simulink model "Dynamic"  (R2016b)
settings: Solver=ode4  StartTime=0.0  StopTime=13.7777  FixedStep=0.01  RelTol=1e-3
settings Model: Creator=Admin  LastModifiedBy=HP

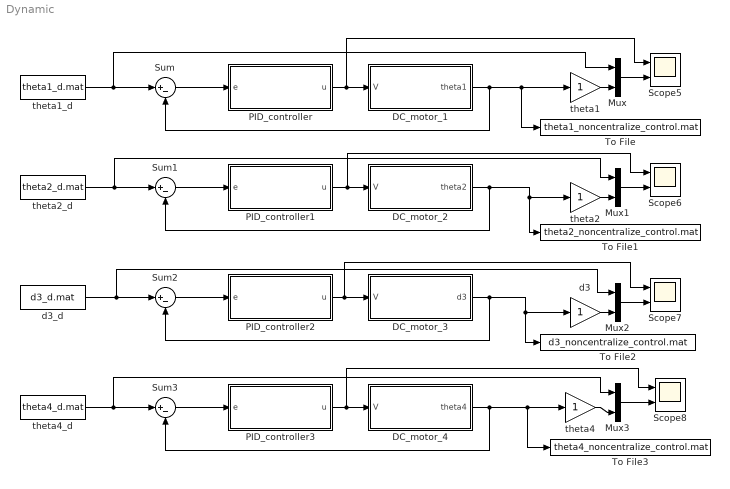
== system Dynamic ==
  DC_motor_1 : Subsystem  mask{Ki=0.1, Kb=0.1, L=0.5, R=2.0, Jeff=0.02, Beff=0.2, N=200}
  DC_motor_2 : Subsystem  mask{Ki=0.1, Kb=0.1, L=0.5, R=2.0, Jeff=0.02, Beff=0.2, N=100}
  DC_motor_3 : Subsystem  mask{Ki=0.1, Kb=0.1, L=0.5, R=2.0, Jeff=0.02, Beff=0.2, N=100}
  DC_motor_4 : Subsystem  mask{Ki=0.1, Kb=0.1, L=0.5, R=2.0, Jeff=0.02, Beff=0.2, N=50}
  Mux{,1..3} (4 alike) : Mux  Inputs=2
  PID_controller : Subsystem  mask{Kp=60000, Ki=8000, Kd=8000}
  PID_controller1 : Subsystem  mask{Kp=30000, Ki=4000, Kd=4000}
  PID_controller2 : Subsystem  mask{Kp=30000, Ki=4000, Kd=4000}
  PID_controller3 : Subsystem  mask{Kp=10000, Ki=2000, Kd=2000}
  Scope{5..8} (4 alike) : Scope  NumInputPorts=2
  Sum{,1..3} (4 alike) : Sum  Inputs=|+-
  To File : ToFile  Filename=theta1_noncentralize_control.mat  MatrixName=theta1_noncentralize_control
  To File1 : ToFile  Filename=theta2_noncentralize_control.mat  MatrixName=theta2_noncentralize_control
  To File2 : ToFile  Filename=d3_noncentralize_control.mat  MatrixName=d3_noncentralize_control
  To File3 : ToFile  Filename=theta4_noncentralize_control.mat  MatrixName=theta4_noncentralize_control
  d3 : Gain
  d3_d : FromFile  FileName=d3_d.mat  SampleTime=0
  theta1 : Gain
  theta1_d : FromFile  FileName=theta1_d.mat  SampleTime=0
  theta2 : Gain
  theta2_d : FromFile  FileName=theta2_d.mat  SampleTime=0
  theta4 : Gain
  theta4_d : FromFile  FileName=theta4_d.mat  SampleTime=0
  wires:
  DC_motor_1/1(theta1) -> Sum/2, To File/1, theta1/1
  Sum/1 -> PID_controller/1(e)
  PID_controller/1(u) -> Scope5/1, DC_motor_1/1(V)
  DC_motor_2/1(theta2) -> Sum1/2, To File1/1, theta2/1
  Sum1/1 -> PID_controller1/1(e)
  PID_controller1/1(u) -> Scope6/1, DC_motor_2/1(V)
  Sum2/1 -> PID_controller2/1(e)
  PID_controller2/1(u) -> Scope7/1, DC_motor_3/1(V)
  DC_motor_4/1(theta4) -> Sum3/2, To File3/1, theta4/1
  Sum3/1 -> PID_controller3/1(e)
  PID_controller3/1(u) -> Scope8/1, DC_motor_4/1(V)
  theta1_d/1 -> Mux/1, Sum/1
  DC_motor_3/1(d3) -> Sum2/2, To File2/1, d3/1
  theta2_d/1 -> Mux1/1, Sum1/1
  d3_d/1 -> Mux2/1, Sum2/1
  theta4_d/1 -> Mux3/1, Sum3/1
  theta1/1 -> Mux/2
  theta2/1 -> Mux1/2
  d3/1 -> Mux2/2
  theta4/1 -> Mux3/2
  Mux/1 -> Scope5/2
  Mux1/1 -> Scope6/2
  Mux2/1 -> Scope7/2
  Mux3/1 -> Scope8/2

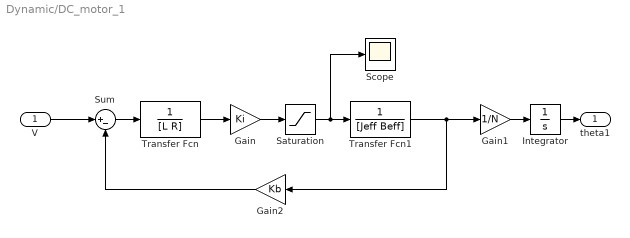
== system Dynamic/DC_motor_1 ==
  V : Inport
  Gain : Gain  Gain=Ki
  Gain1 : Gain  Gain=1/N
  Gain2 : Gain  Gain=Kb
  Integrator : Integrator  InitialCondition=-1.8171
  Saturation : Saturate  UpperLimit=10000  LowerLimit=-10000
  Scope : Scope
  Sum : Sum  Inputs=|+-
  Transfer Fcn : TransferFcn  Denominator=[L R]
  Transfer Fcn1 : TransferFcn  Denominator=[Jeff Beff]
  theta1 : Outport
  wires:
  Sum/1 -> Transfer Fcn/1
  Transfer Fcn/1 -> Gain/1
  Gain/1 -> Saturation/1
  Transfer Fcn1/1 -> Gain1/1, Gain2/1
  Gain2/1 -> Sum/2
  V/1 -> Sum/1
  Saturation/1 -> Scope/1, Transfer Fcn1/1
  Gain1/1 -> Integrator/1
  Integrator/1 -> theta1/1

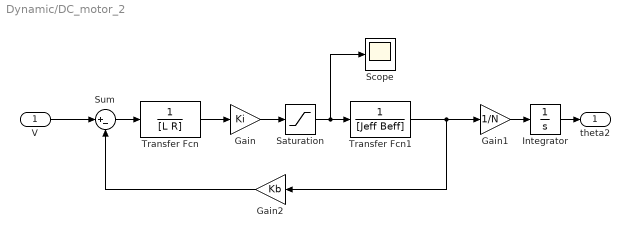
== system Dynamic/DC_motor_2 ==
  V : Inport
  Gain : Gain  Gain=Ki
  Gain1 : Gain  Gain=1/N
  Gain2 : Gain  Gain=Kb
  Integrator : Integrator  InitialCondition=-1.1709
  Saturation : Saturate  UpperLimit=10000  LowerLimit=-10000
  Scope : Scope
  Sum : Sum  Inputs=|+-
  Transfer Fcn : TransferFcn  Denominator=[L R]
  Transfer Fcn1 : TransferFcn  Denominator=[Jeff Beff]
  theta2 : Outport
  wires:
  Sum/1 -> Transfer Fcn/1
  Transfer Fcn/1 -> Gain/1
  Gain/1 -> Saturation/1
  Transfer Fcn1/1 -> Gain1/1, Gain2/1
  Gain2/1 -> Sum/2
  V/1 -> Sum/1
  Saturation/1 -> Scope/1, Transfer Fcn1/1
  Gain1/1 -> Integrator/1
  Integrator/1 -> theta2/1

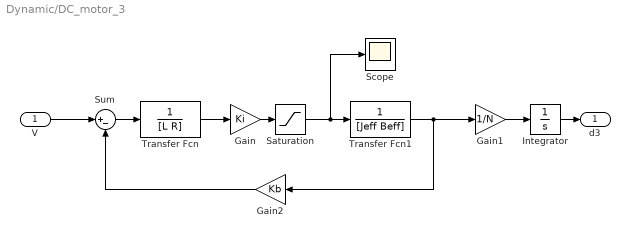
== system Dynamic/DC_motor_3 ==
  V : Inport
  Gain : Gain  Gain=Ki
  Gain1 : Gain  Gain=1/N
  Gain2 : Gain  Gain=Kb
  Integrator : Integrator
  Saturation : Saturate  UpperLimit=10000  LowerLimit=-10000
  Scope : Scope
  Sum : Sum  Inputs=|+-
  Transfer Fcn : TransferFcn  Denominator=[L R]
  Transfer Fcn1 : TransferFcn  Denominator=[Jeff Beff]
  d3 : Outport
  wires:
  Sum/1 -> Transfer Fcn/1
  Transfer Fcn/1 -> Gain/1
  Gain/1 -> Saturation/1
  Transfer Fcn1/1 -> Gain1/1, Gain2/1
  Gain2/1 -> Sum/2
  V/1 -> Sum/1
  Saturation/1 -> Scope/1, Transfer Fcn1/1
  Gain1/1 -> Integrator/1
  Integrator/1 -> d3/1

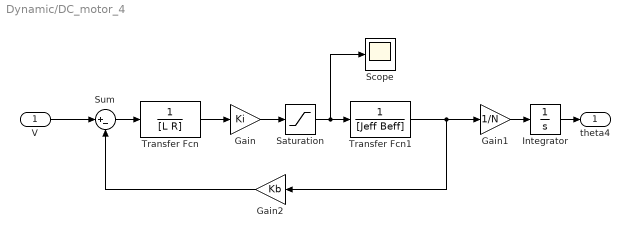
== system Dynamic/DC_motor_4 ==
  V : Inport
  Gain : Gain  Gain=Ki
  Gain1 : Gain  Gain=1/N
  Gain2 : Gain  Gain=Kb
  Integrator : Integrator  InitialCondition=-1.7257
  Saturation : Saturate  UpperLimit=10000  LowerLimit=-10000
  Scope : Scope
  Sum : Sum  Inputs=|+-
  Transfer Fcn : TransferFcn  Denominator=[L R]
  Transfer Fcn1 : TransferFcn  Denominator=[Jeff Beff]
  theta4 : Outport
  wires:
  Sum/1 -> Transfer Fcn/1
  Transfer Fcn/1 -> Gain/1
  Gain/1 -> Saturation/1
  Transfer Fcn1/1 -> Gain1/1, Gain2/1
  Gain2/1 -> Sum/2
  V/1 -> Sum/1
  Saturation/1 -> Scope/1, Transfer Fcn1/1
  Gain1/1 -> Integrator/1
  Integrator/1 -> theta4/1

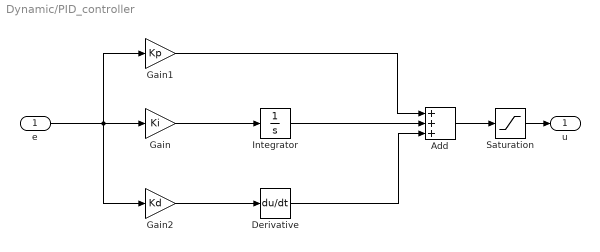
== system Dynamic/PID_controller ==
  e : Inport
  Add : Sum  Inputs=+++
  Derivative : Derivative
  Gain : Gain  Gain=Ki
  Gain1 : Gain  Gain=Kp
  Gain2 : Gain  Gain=Kd
  Integrator : Integrator
  Saturation : Saturate  UpperLimit=300  LowerLimit=-300
  u : Outport
  wires:
  e/1 -> Gain2/1, Gain1/1, Gain/1
  Gain/1 -> Integrator/1
  Gain2/1 -> Derivative/1
  Gain1/1 -> Add/1
  Integrator/1 -> Add/2
  Derivative/1 -> Add/3
  Add/1 -> Saturation/1
  Saturation/1 -> u/1

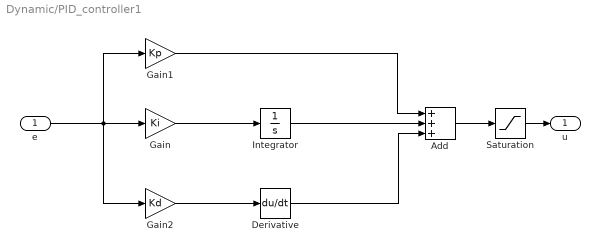
== system Dynamic/PID_controller1 ==
  e : Inport
  Add : Sum  Inputs=+++
  Derivative : Derivative
  Gain : Gain  Gain=Ki
  Gain1 : Gain  Gain=Kp
  Gain2 : Gain  Gain=Kd
  Integrator : Integrator
  Saturation : Saturate  UpperLimit=200  LowerLimit=-200
  u : Outport
  wires:
  e/1 -> Gain2/1, Gain1/1, Gain/1
  Gain/1 -> Integrator/1
  Gain2/1 -> Derivative/1
  Gain1/1 -> Add/1
  Integrator/1 -> Add/2
  Derivative/1 -> Add/3
  Add/1 -> Saturation/1
  Saturation/1 -> u/1

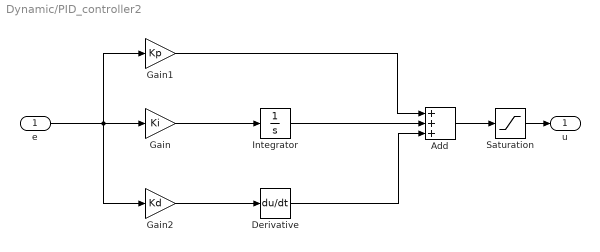
== system Dynamic/PID_controller2 ==
  e : Inport
  Add : Sum  Inputs=+++
  Derivative : Derivative
  Gain : Gain  Gain=Ki
  Gain1 : Gain  Gain=Kp
  Gain2 : Gain  Gain=Kd
  Integrator : Integrator
  Saturation : Saturate  UpperLimit=200  LowerLimit=-200
  u : Outport
  wires:
  e/1 -> Gain2/1, Gain1/1, Gain/1
  Gain/1 -> Integrator/1
  Gain2/1 -> Derivative/1
  Gain1/1 -> Add/1
  Integrator/1 -> Add/2
  Derivative/1 -> Add/3
  Add/1 -> Saturation/1
  Saturation/1 -> u/1

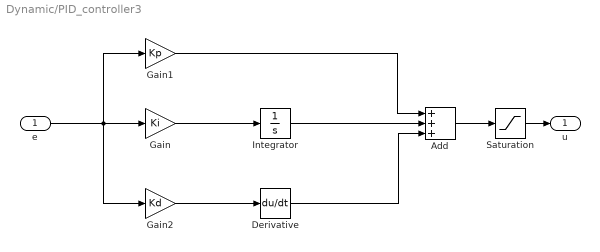
== system Dynamic/PID_controller3 ==
  e : Inport
  Add : Sum  Inputs=+++
  Derivative : Derivative
  Gain : Gain  Gain=Ki
  Gain1 : Gain  Gain=Kp
  Gain2 : Gain  Gain=Kd
  Integrator : Integrator
  Saturation : Saturate  UpperLimit=100  LowerLimit=-100
  u : Outport
  wires:
  e/1 -> Gain2/1, Gain1/1, Gain/1
  Gain/1 -> Integrator/1
  Gain2/1 -> Derivative/1
  Gain1/1 -> Add/1
  Integrator/1 -> Add/2
  Derivative/1 -> Add/3
  Add/1 -> Saturation/1
  Saturation/1 -> u/1
